simulink model "PROB1"  (R2020a)
settings: Solver=VariableStepAuto  StartTime=0.0  StopTime=10.0  RelTol=1e-3
model workspace (MAT data in the model file):
  B = Simulink.Parameter
  B.Value = 50
  B.DataType = 'auto'
  B.Dimensions = [1 1]
  K1 = Simulink.Parameter
  K1.Value = 50
  K1.DataType = 'auto'
  K1.Dimensions = [1 1]
  K12 = Simulink.Parameter
  K12.Value = 100
  K12.DataType = 'auto'
  K12.Dimensions = [1 1]
  M1 = Simulink.Parameter
  M1.Value = 100
  M1.DataType = 'auto'
  M1.Dimensions = [1 1]
  M2 = Simulink.Parameter
  M2.Value = 100
  M2.DataType = 'auto'
  M2.Dimensions = [1 1]
  PI = Simulink.Parameter
  PI.Value = 3.14
  PI.DataType = 'auto'
  PI.Dimensions = [1 1]
settings Model: Creator=akhil singh  LastModifiedBy=akhil singh

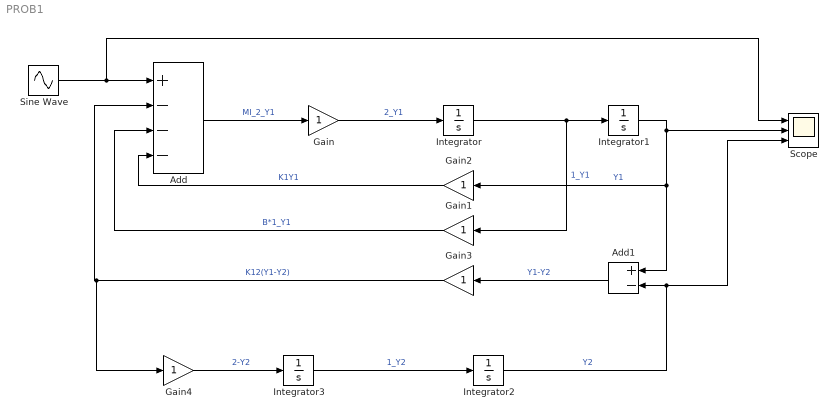
== system PROB1 ==
  Add : Sum  Inputs=+---
  Add1 : Sum  Inputs=+-
  Gain{,1..4} (5 alike) : Gain
  Integrator{,1..3} (4 alike) : Integrator
  Scope : Scope  NumInputPorts=3
  Sine Wave : Sin  Amplitude=10  Frequency=10*2*PI  SampleTime=0
  wires:
  Sine Wave/1 -> Scope/1, Add/1
  Add/1 -> Gain/1  "MI_2_Y1"
  Gain4/1 -> Integrator3/1  "2-Y2"
  Integrator3/1 -> Integrator2/1  "1_Y2"
  Gain/1 -> Integrator/1  "2_Y1"
  Integrator/1 -> Gain1/1, Integrator1/1  "1_Y1"
  Integrator1/1 -> Gain2/1, Add1/1, Scope/2  "Y1"
  Add1/1 -> Gain3/1  "Y1-Y2"
  Integrator2/1 -> Scope/3, Add1/2  "Y2"
  Gain2/1 -> Add/4  "K1Y1"
  Gain1/1 -> Add/3  "B*1_Y1"
  Gain3/1 -> Gain4/1, Add/2  "K12(Y1-Y2)"
